simulink model "final"  (R2020b)
settings: Solver=FixedStepDiscrete  StartTime=0.0  StopTime=inf  FixedStep=0.01  RelTol=1e-3
undefined symbols (not defined in the file or in its folder): motorIp, motorSp
libraries: mobileRoboticsTrainingLib x5, fuzblock x1
settings Model: Creator=DAMFODUM  LastModifiedBy=DAMFODUM

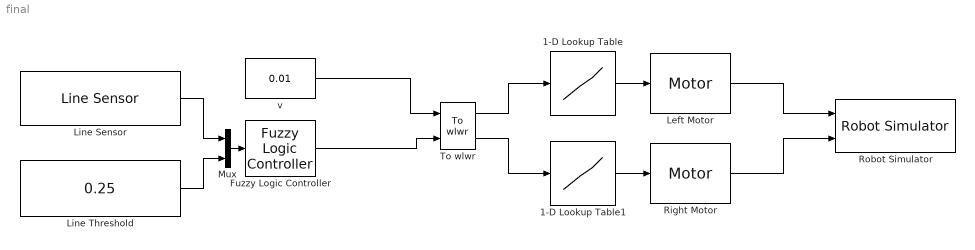
== system final ==
  1-D Lookup Table : Lookup_n-D  NumberOfTableDimensions=1  BreakpointsForDimension1=motorSp  Table=motorIp  ExtrapMethod=Clip  InternalRulePriority=Speed  RndMeth=Simplest  InputSameDT=on
  1-D Lookup Table1 : Lookup_n-D  NumberOfTableDimensions=1  BreakpointsForDimension1=motorSp  Table=motorIp  ExtrapMethod=Clip  InternalRulePriority=Speed  RndMeth=Simplest  InputSameDT=on
  Fuzzy Logic Controller : fuzblock/Fuzzy Logic  Controller  FIS='FTEST.fis'  OutputSampleNumber=101  DataType=double  FuzzifiedInputs=off  RuleFiringStrengths=off  RuleOutputs=off  AggregatedOutputs=off  SimulateUsing=Interpreted execution  OutOfRangeInputValueMessage=warning  NoRuleFiredMessage=warning  EmptyOutputFuzzySetMessage=warning
  Left Motor : mobileRoboticsTrainingLib/Motor  motorPlant=wheelMotorModel  sensorType=Speed
      settings: SourceProductName=Mobile Robotics Training Library
  Line Sensor : mobileRoboticsTrainingLib/Line Sensor  mapVariable=mapForSim  envVal=1  lineVal=-1  sensOff=[0.01 0]
      settings: SourceProductName=Mobile Robotics Training Library
  Line Threshold : Constant  Value=0.25
  Mux : Mux  Inputs=2
  Right Motor : mobileRoboticsTrainingLib/Motor  motorPlant=wheelMotorModel  sensorType=Speed
      settings: SourceProductName=Mobile Robotics Training Library
  Robot Simulator : mobileRoboticsTrainingLib/Robot Simulator  Priority=99  mapVar=mapForSim  startX=0.25346  startY=0.73445  startTheta=0  axleLength=axleLength  wheelR=wheelR
  To wlwr : mobileRoboticsTrainingLib/To wlwr  axleLength=axleLength  wheelR=wheelR
  v : Constant  Value=0.01
  wires:
  Line Threshold/1 -> Mux/2
  Fuzzy Logic Controller/1 -> To wlwr/2
  Right Motor/1 -> Robot Simulator/2
  To wlwr/2 -> 1-D Lookup Table1/1
  Line Sensor/1 -> Mux/1
  v/1 -> To wlwr/1
  1-D Lookup Table/1 -> Left Motor/1
  To wlwr/1 -> 1-D Lookup Table/1
  1-D Lookup Table1/1 -> Right Motor/1
  Left Motor/1 -> Robot Simulator/1
  Mux/1 -> Fuzzy Logic Controller/1
